simulink subsystem "Encoders"  (R2024a)
settings: Solver=VariableStepAuto  StartTime=0.0  StopTime=10.0  RelTol=1e-3
model mask{bit_resolution=0, bit_noise=0, seed=0, Ts=0}
  mask prompts: bit_resolution "Bits of resolution"; bit_noise "Bits of noise"; Ts "Sample time (s)"
settings Model: Creator=upattacini  LastModifiedBy=upattacini

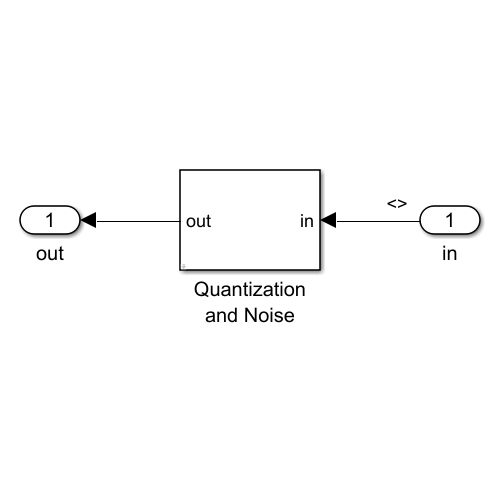
[thumbnail: Simulink's stored preview of the top-level diagram]
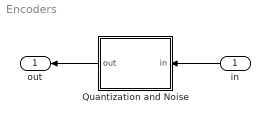
== system Encoders ==
  in : Inport
  Quantization and Noise : Subsystem  mask{bit_resolution=bit_resolution, bit_noise=bit_noise, seed=0, Ts=Ts}
      mask prompts: bit_resolution "Resolution bits"; bit_noise "Noise bits"; Ts "Sample time (s)"
      settings: PortSchema="{\"entries\":[{\"content\":{\"sides\":[{\"content\":{\"connectorIds\":[\"Out1\"]},\"type\":\"ConnectorPlacement.EquallySpacedRectSide\",\"uuid\":\"5c60203e-1477-4c63-bf85-2a9264896243\"},{\"content\":{\"connectorIds\":[\"In1\"],\"side\":\"RIGHT\"},\"type\":\"ConnectorPlacement.EquallySpacedRectSide\",\"uuid\":\"fde9215e-0eee-4b90-b3d3-bc5e0578faf0\"},{\"content\":{\"side\":\"TOP\"},\"type\":\"ConnectorPlacement.EquallySpacedRectSide\",\"uuid\":\"75472767-9856-4b99-a0f4-bd856ef58e73\"}]},\"type\":\"ConnectorPlacement.EquallySpacedConnector\",\"uuid\":\"089ac2bf-9317-43ab-ab34-2d9e1bbbe948\"}],\"packageUris\":[\"http://schema.mathworks.com/mf0/Connector/R2020b\"],\"version\":\"1.0\"}"
  out : Outport
  wires:
  in/1 -> Quantization and Noise/1(in)
  Quantization and Noise/1(out) -> out/1

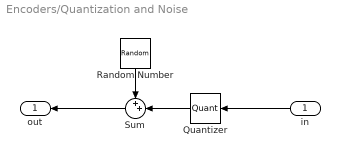
== system Encoders/Quantization and Noise ==
  in : Inport
  Quantizer : Quantizer  QuantizationInterval=360/2^bit_resolution
  Random Number : RandomNumber  Variance=(360/2^(bit_resolution-bit_noise) * 0.25)^2  Seed=seed  SampleTime=Ts
  Sum : Sum  Inputs=++|
  out : Outport
  wires:
  Quantizer/1 -> Sum/2
  Random Number/1 -> Sum/1
  in/1 -> Quantizer/1
  Sum/1 -> out/1
